simulink library "Lib_PMSMCtrl_2016b"  (R2016b)
settings: Solver=VariableStepAuto  StartTime=0.0  StopTime=10.0  RelTol=1e-3
libraries: mcbcontrolslib x1
settings Model: Creator=62555  LastModifiedBy=62555
settings DataIOCC: ReturnWorkspaceOutputs=on
settings DebuggingCC: UnconnectedInputMsg=none  UnconnectedOutputMsg=none  UnconnectedLineMsg=none
settings ModelReferenceCC: EnableRefExpFcnMdlSchedulingChecks=off
settings SFSimCC: SimUseLocalCustomCode=on
settings RTWCC: RTWUseLocalCustomCode=on

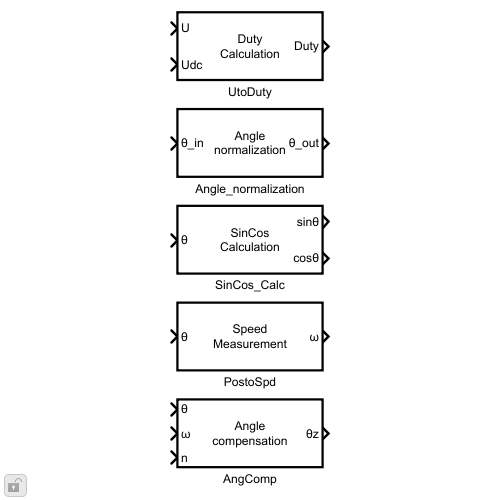
[thumbnail: Simulink's stored preview of the top-level diagram]
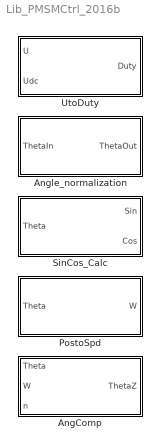
== system Lib_PMSMCtrl_2016b ==
  AngComp : Subsystem  TreatAsAtomicUnit=on  RTWFileName=Lib_PMSMCtrl  mask{Ts=0}
      settings: RTWFcnNameOpts=Use subsystem name  RTWFileNameOpts=User specified
      mask Display:
      | port_label('input', 1, 'θ');
      | port_label('input', 2, 'ω');
      | port_label('input', 3, 'n');
      | port_label('output', 1, 'θz');
      | disp('Angle\ncompensation');
  Angle_normalization : MATLAB Function  TreatAsAtomicUnit=on
  PostoSpd : Subsystem  TreatAsAtomicUnit=on  RTWFileName=Lib_PMSMCtrl  mask{Ts=1}
      settings: RTWFcnNameOpts=Use subsystem name  RTWFileNameOpts=User specified
      mask Display:
      | disp('Speed\nMeasurement');
      | 
      | 
      | %disp('Speed Measurement');
      | port_label('input', 1, 'θ');
      | port_label('output', 1, 'ω');
  SinCos_Calc : Subsystem  TreatAsAtomicUnit=on  RTWFileName=Lib_PMSMCtrl
      settings: RTWFcnNameOpts=Use subsystem name  RTWFileNameOpts=User specified
      mask Display:
      | disp('SinCos\nCalculation');
      | port_label('input', 1, 'θ');
      | port_label('output', 1, 'sinθ');
      | port_label('output', 2, 'cosθ');
  UtoDuty : Subsystem  TreatAsAtomicUnit=on  RTWFileName=Lib_PMSMCtrl
      settings: RTWFcnNameOpts=Use subsystem name  RTWFileNameOpts=User specified
      mask Display:
      | disp('Duty\nCalculation');
      | port_label('input', 1, 'U');
      | port_label('input', 2, 'Udc');
      | port_label('output', 1, 'Duty');

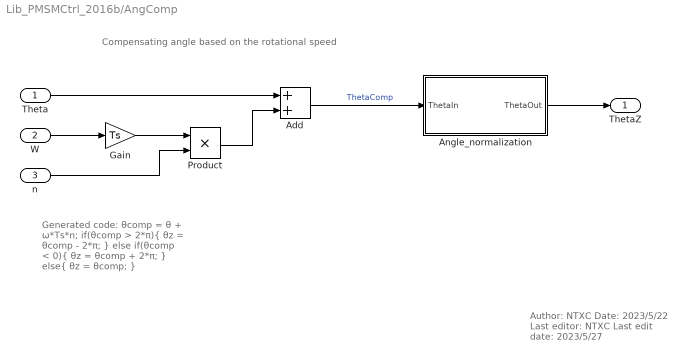
== system Lib_PMSMCtrl_2016b/AngComp ==
  note: Compensating angle based on the rotational speed
  note: Generated code:
      |
      | θcomp = θ + ω*Ts*n;
      |
      | if(θcomp > 2*π){
      |     θz = θcomp - 2*π;
      | } else if(θcomp < 0){
      |     θz = θcomp + 2*π;
      | } else{
      |     θz = θcomp;
      | }
  note: Author: NTXC
      | Date: 2023/5/22
      | Last editor: NTXC
      | Last edit date: 2023/5/27
  Theta : Inport
  W : Inport  Port=2
  n : Inport  Port=3
  Add : Sum
  Angle_normalization : MATLAB Function  TreatAsAtomicUnit=on
  Gain : Gain  Gain=Ts
  Product : Product
  ThetaZ : Outport
  wires:
  Add/1 -> Angle_normalization/1(ThetaIn)  "ThetaComp"
  Gain/1 -> Product/1
  W/1 -> Gain/1
  Theta/1 -> Add/1
  Product/1 -> Add/2
  n/1 -> Product/2
  Angle_normalization/1(ThetaOut) -> ThetaZ/1

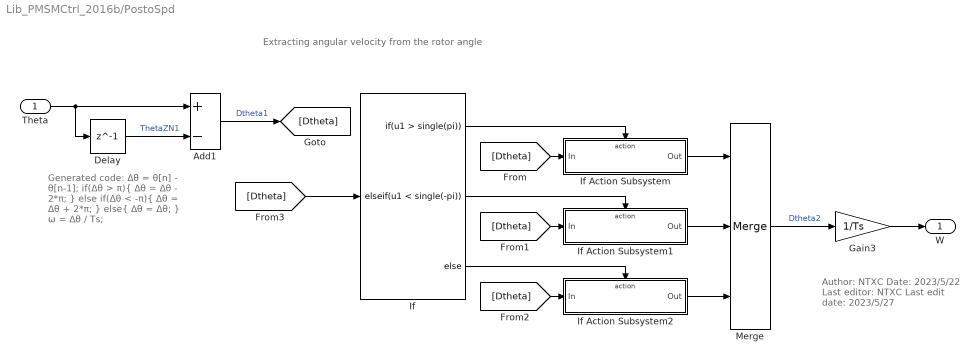
== system Lib_PMSMCtrl_2016b/PostoSpd ==
  note: Generated code:
      |
      | Δθ = θ[n] - θ[n-1];
      | if(Δθ > π){
      |     Δθ = Δθ - 2*π;
      | } else if(Δθ < -π){
      |     Δθ = Δθ + 2*π;
      | } else{
      |     Δθ = Δθ;
      | }
      |
      | ω = Δθ / Ts;
  note: Author: NTXC
      | Date: 2023/5/22
      | Last editor: NTXC
      | Last edit date: 2023/5/27
  note: Extracting angular velocity from the rotor angle
  Theta : Inport
  Add1 : Sum  Inputs=+-
  Delay : Delay  DelayLength=1
  Gain3 : Gain  Gain=1/Ts
  If : If  IfExpression=u1 > single(pi)  ElseIfExpressions=u1 < single(-pi)
  If Action Subsystem : Subsystem  TreatAsAtomicUnit=on
  If Action Subsystem1 : Subsystem  TreatAsAtomicUnit=on
  If Action Subsystem2 : Subsystem  TreatAsAtomicUnit=on
  Merge : Merge  Inputs=3
  W : Outport
  wires:
  If Action Subsystem2/1(Out) -> Merge/3
  If Action Subsystem1/1(Out) -> Merge/2
  If Action Subsystem/1(Out) -> Merge/1
  Delay/1 -> Add1/2  "ThetaZN1"
  Theta/1 -> Delay/1, Add1/1
  Merge/1 -> Gain3/1  "Dtheta2"
  Gain3/1 -> W/1
  If/1 -> If Action Subsystem/Action
  If/2 -> If Action Subsystem1/Action
  If/3 -> If Action Subsystem2/Action
  [Dtheta] -> If Action Subsystem/1(In)
  [Dtheta] -> If Action Subsystem1/1(In)
  [Dtheta] -> If Action Subsystem2/1(In)
  Add1/1 -> [Dtheta]  "Dtheta1"
  [Dtheta] -> If/1

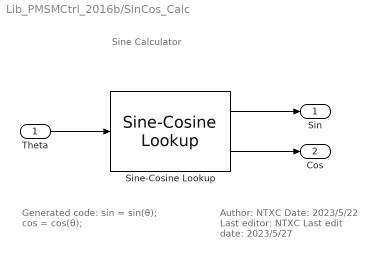
== system Lib_PMSMCtrl_2016b/SinCos_Calc ==
  note: Author: NTXC
      | Date: 2023/5/22
      | Last editor: NTXC
      | Last edit date: 2023/5/27
  note: Sine Calculator
  note: Generated code:
      |
      | sin = sin(θ);
      | cos = cos(θ);
  Theta : Inport
  Sine-Cosine Lookup : mcbcontrolslib/Sine-Cosine Lookup  AngleInput=Radians  N_points=4095
  Sin : Outport
  Cos : Outport  Port=2
  wires:
  Theta/1 -> Sine-Cosine Lookup/1
  Sine-Cosine Lookup/1 -> Sin/1
  Sine-Cosine Lookup/2 -> Cos/1

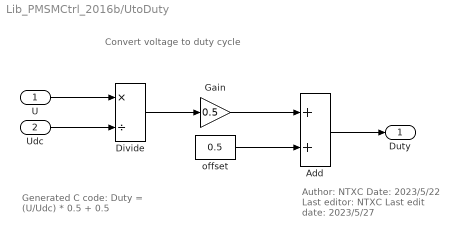
== system Lib_PMSMCtrl_2016b/UtoDuty ==
  note: Convert voltage to duty cycle
  note: Generated C code:
      |
      | Duty = (U/Udc) * 0.5 + 0.5
  note: Author: NTXC
      | Date: 2023/5/22
      | Last editor: NTXC
      | Last edit date: 2023/5/27
  U : Inport
  Udc : Inport  Port=2
  Add : Sum
  Divide : Product  Inputs=*/
  Gain : Gain  Gain=0.5
  offset : Constant  Value=0.5  OutDataTypeStr=single  SampleTime=-1
  Duty : Outport
  wires:
  Divide/1 -> Gain/1
  Gain/1 -> Add/1
  offset/1 -> Add/2
  U/1 -> Divide/1
  Add/1 -> Duty/1
  Udc/1 -> Divide/2

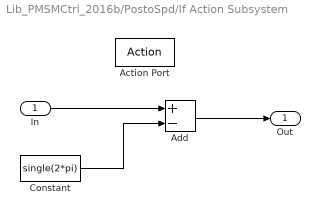
== system Lib_PMSMCtrl_2016b/PostoSpd/If Action Subsystem ==
  In : Inport
  Action Port : ActionPort
  Add : Sum  Inputs=+-
  Constant : Constant  Value=single(2*pi)  OutDataTypeStr=single  SampleTime=-1
  Out : Outport
  wires:
  In/1 -> Add/1
  Add/1 -> Out/1
  Constant/1 -> Add/2

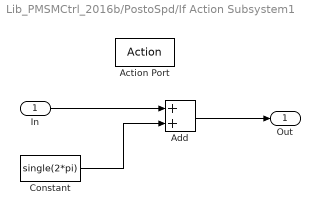
== system Lib_PMSMCtrl_2016b/PostoSpd/If Action Subsystem1 ==
  In : Inport
  Action Port : ActionPort
  Add : Sum
  Constant : Constant  Value=single(2*pi)  OutDataTypeStr=single  SampleTime=-1
  Out : Outport
  wires:
  In/1 -> Add/1
  Constant/1 -> Add/2
  Add/1 -> Out/1

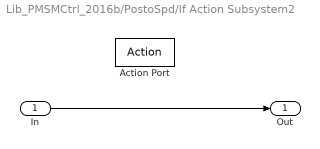
== system Lib_PMSMCtrl_2016b/PostoSpd/If Action Subsystem2 ==
  In : Inport
  Action Port : ActionPort
  Out : Outport
  wires:
  In/1 -> Out/1

== matlab function Lib_PMSMCtrl_2016b/AngComp/Angle_normalization ==
  data: ThetaIn input; ThetaOut output
function ThetaOut = fcn(ThetaIn)

% Author: NTXC
% Date: 2023/5/22
% Last editor: NTXC
% Last edit date: 2023/5/27
%
% Description: Normalize any angle value to the range of 0 to 2π.

Theta = ThetaIn;

while(Theta > single(2*pi))
    Theta = Theta - single(2*pi);
end

while(Theta < single(0))
    Theta = Theta + single(2*pi);
end

ThetaOut = Theta;

== matlab function Lib_PMSMCtrl_2016b/Angle_normalization ==
  data: ThetaIn input; ThetaOut output
function ThetaOut = fcn(ThetaIn)

% Author: NTXC
% Date: 2023/5/22
% Last editor: NTXC
% Last edit date: 2023/5/27
%
% Description: Normalize any angle value to the range of 0 to 2π.

Theta = ThetaIn;

while(Theta > single(2*pi))
    Theta = Theta - single(2*pi);
end

while(Theta < single(0))
    Theta = Theta + single(2*pi);
end

ThetaOut = Theta;
